simulink library "aeroSurface_ul"  (R2018b)
settings: Solver=VariableStepAuto  StartTime=0.0  StopTime=10.0  RelTol=1e-3
values from neighbouring files (symbols this model uses):
  aeroTable = loadAeroTable(airfoilSelectionObj.Value,     clFitLims,clFitOrder,cdFitLims,cdFitOrder,OE,AR,useFit)    [setAirfoilCallback.m]
  RBody2Surf = [xUnitVec(:)';      yUnitVec(:)';      zUnitvec(:)']    [aeroSurface_init.m]
  RSurf2Body = inv(RBody2Surf)    [aeroSurface_init.m]
libraries: vrlib x3
settings Model: Creator=mcobb  LastModifiedBy=mcobb

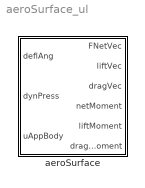
== system aeroSurface_ul ==
  aeroSurface : Subsystem  mask{rAeroCent=[1 0 0], uSpan=[0 1 0], uChord=[0 0 1], airfoilSelection=NACA 2415_T1_Re5.085_M0.00_N9.0.txt, ARef=1, AR=8, OE=0.8, useFit=on, clFitLims=[-10 10], clFitOrder=1, cdFitLims=[-10 10], cdFitOrder=2}
      mask prompts: rAeroCent "Aerodynamic center position vector"; uSpan "Spanwise positive rotation unit vector"; uChord "Increasing chord direction in body frame unit vector"; airfoilSelection "Airfoil"; ARef "Reference area"; AR "Aspect ratio"; OE "Oswald efficiency"; useFit "Use Best Fit Data"; clFitLims "CL fit range (deg) [Lower Upper]"; clFitOrder "CL Fit Order"; cdFitLims "CD fit range (deg) [Lower Upper]"; cdFitOrder "CD Fit Oder"
      mask help:
      | Block to model a generic planar aerodynamic surface that rotates about its span.
      |
      | Note that all vectors are in the body fixed coordinate system and are relative to the origin of that coordinate system (which is probably the center of mass).
      |
      | Click the help button for more details on the spanwise positive rotation vector.
      |
      | 5/14/19
      | -MC
      mask init:
      | aeroSurface_init
      mask Help: One of the inputs to this block is the spanwise positive rotation vector.  This is the vector that define exactly what constitutes a positive or negative deflection of the control surface.  If the signal into the deflAng is positive, it is interpreted to mean that this planar surface is rotated by that amount about this unit vector.
      mask TypeOptions airfoilSelection: NACA 1408_T1_Re5.085_M0.00_N9.0.txt | NACA 1410_T1_Re5.085_M0.00_N9.0.txt | NACA 2.5411_T1_Re5.085_M0.00_N9.0.txt | NACA 2408_T1_Re5.085_M0.00_N9.0.txt | NACA 2410_T1_Re5.085_M0.00_N9.0.txt | NACA 2412_T1_Re5.085_M0.00_N9.0.txt | NACA 2415_T1_Re5.085_M0.00_N9.0.txt | NACA 2418_T1_Re5.085_M0.00_N9.0.txt | NACA 2421_T1_Re5.085_M0.00_N9.0.txt | NACA 2424_T1_Re5.085_M0.00_N9.0.txt | NACA 4412_T1_Re5.085_M0.00_N9.0.txt | NACA 4415_T1_Re5.085_M0.00_N9.0.txt | NACA 4418_T1_Re5.085_M0.00_N9.0.txt | NACA 4421_T1_Re5.085_M0.00_N9.0.txt | NACA 4424_T1_Re5.085_M0.00_N9.0.txt | NACA 6412_T1_Re5.085_M0.00_N9.0.txt | NACA-0009 9.0% smoothed_T1_Re1.000_M0.00_N9.0.txt
      mask Callback airfoilSelection: setAirfoilCallback
      mask Callback useFit: bestFitCoeffDataToggle
      mask DialogControl fitParameterBox Prompt: Fitting Parameters

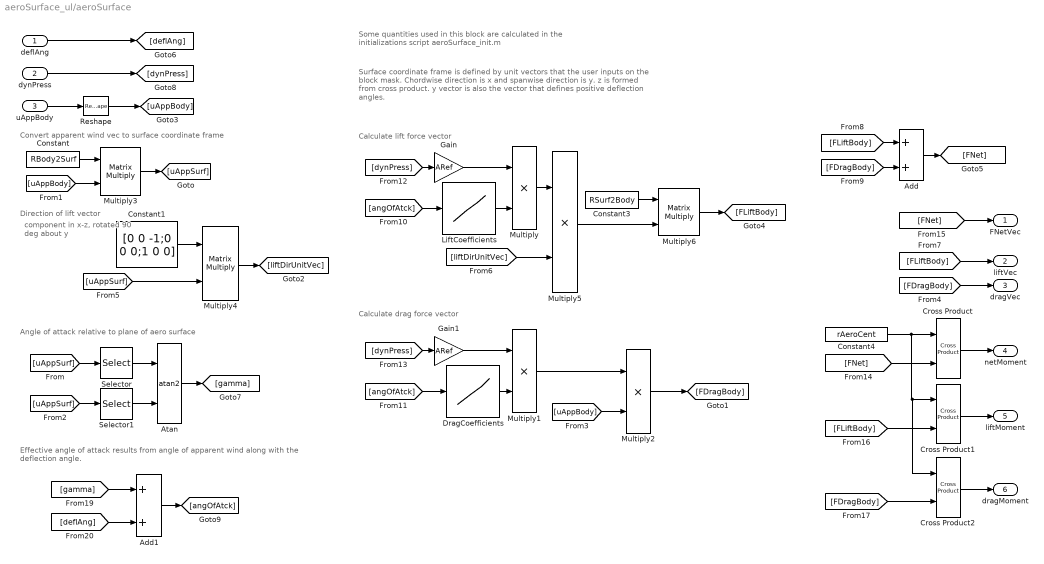
== system aeroSurface_ul/aeroSurface ==
  note: component in x-z,
      | rotated 90 deg
      | about y
  note: Effective angle of attack results from angle of apparent
      | wind along with the deflection angle.
  note: Calculate drag force vector
  note: Calculate lift force vector
  note: Surface coordinate frame is defined by unit vectors that the
      | user inputs on the block mask. Chordwise direction is x and
      | spanwise direction is y. z is formed from cross product. y
      | vector is also the vector that defines positive deflection angles.
  note: Convert apparent wind vec to surface coordinate frame
  note: Direction of lift vector
  note: Angle of attack relative to plane of aero surface
  note: Some quantities used in this block are calculated
      | in the initializations script aeroSurface_init.m
  deflAng : Inport
  dynPress : Inport  Port=2
  uAppBody : Inport  Port=3
  Add : Sum
  Add1 : Sum
  Atan : Trigonometry  Operator=atan2
  Constant : Constant  Value=RBody2Surf
  Constant1 : Constant  Value=[0 0 -1;0 0 0;1 0 0]
  Constant3 : Constant  Value=RSurf2Body
  Constant4 : Constant  Value=rAeroCent
  Cross Product : vrlib/Utilities/Cross Product
      settings: SourceProductBaseCode=VR
  Cross Product1 : vrlib/Utilities/Cross Product
      settings: SourceProductBaseCode=VR
  Cross Product2 : vrlib/Utilities/Cross Product
      settings: SourceProductBaseCode=VR
  DragCoefficients : Lookup_n-D  NumberOfTableDimensions=1  BreakpointsForDimension1=aeroTable.alpha  Table=aeroTable.cd  ExtrapMethod=Clip  UseLastTableValue=on  InternalRulePriority=Speed  RndMeth=Simplest  InputSameDT=on
  Gain : Gain  Gain=ARef
  Gain1 : Gain  Gain=ARef
  LiftCoefficients : Lookup_n-D  NumberOfTableDimensions=1  BreakpointsForDimension1=aeroTable.alpha  Table=aeroTable.cl  ExtrapMethod=Clip  UseLastTableValue=on  InternalRulePriority=Speed  RndMeth=Simplest  InputSameDT=on
  Multiply{,1..2,5} (4 alike) : Product
  Multiply3 : Product  Multiplication=Matrix(*)
  Multiply4 : Product  Multiplication=Matrix(*)
  Multiply6 : Product  Multiplication=Matrix(*)
  Reshape : Reshape  OutputDimensionality=Column vector (2-D)
  Selector : Selector  InputPortWidth=3  IndexOptions=Index vector (dialog)  Indices=3  OutputSizes=1
  Selector1 : Selector  InputPortWidth=3  IndexOptions=Index vector (dialog)  Indices=1  OutputSizes=1
  FNetVec : Outport
  liftVec : Outport  Port=2
  dragVec : Outport  Port=3
  netMoment : Outport  Port=4
  liftMoment : Outport  Port=5
  dragMoment : Outport  Port=6
  wires:
  Add1/1 -> [angOfAtck]
  [deflAng] -> Add1/2
  [gamma] -> Add1/1
  deflAng/1 -> [deflAng]
  [FDragBody] -> Cross Product2/2
  [FLiftBody] -> Cross Product1/2
  Cross Product2/1 -> dragMoment/1
  Constant4/1 -> Cross Product/1, Cross Product1/1, Cross Product2/1
  Cross Product1/1 -> liftMoment/1
  [FNet] -> Cross Product/2
  Cross Product/1 -> netMoment/1
  [FNet] -> FNetVec/1
  [FDragBody] -> Add/2
  [FLiftBody] -> Add/1
  Add/1 -> [FNet]
  [FLiftBody] -> liftVec/1
  Multiply6/1 -> [FLiftBody]
  Constant3/1 -> Multiply6/1
  Multiply5/1 -> Multiply6/2
  Multiply/1 -> Multiply5/1
  [liftDirUnitVec] -> Multiply5/2
  Multiply4/1 -> [liftDirUnitVec]
  [uAppSurf] -> Multiply4/2
  [FDragBody] -> dragVec/1
  Multiply2/1 -> [FDragBody]
  [uAppSurf] -> Selector1/1
  [uAppSurf] -> Selector/1
  Multiply3/1 -> [uAppSurf]
  Constant/1 -> Multiply3/1
  [uAppBody] -> Multiply3/2
  Multiply1/1 -> Multiply2/1
  [uAppBody] -> Multiply2/2
  DragCoefficients/1 -> Multiply1/2
  [dynPress] -> Gain1/1
  Gain1/1 -> Multiply1/1
  Gain/1 -> Multiply/1
  LiftCoefficients/1 -> Multiply/2
  [dynPress] -> Gain/1
  [angOfAtck] -> DragCoefficients/1
  [angOfAtck] -> LiftCoefficients/1
  Atan/1 -> [gamma]
  Selector1/1 -> Atan/2
  Selector/1 -> Atan/1
  uAppBody/1 -> Reshape/1
  dynPress/1 -> [dynPress]
  Constant1/1 -> Multiply4/1
  Reshape/1 -> [uAppBody]
